simulink model "Buck_DCM_Model_eZdsp"  (R2020a)
settings: Solver=FixedStepAuto  StartTime=0.0  StopTime=inf  FixedStep=T  RelTol=1e-3
undefined symbols (not defined in the file): C, ILmax, Iumax, J, Kphi, L, Lu, rL, Ru, T, Ubat, Ucmax, wmax
libraries: c280xlib x16, simulink x4, c2833xlib x1
settings Model: SILPILModeSetting=veronly  ExtModeTrigDuration=8  Creator=Nguyen Tung  LastModifiedBy=Nguyen Tung
settings OptimizationCC: DefaultUnderspecifiedDataType=single  StrengthReduction=on  PassReuseOutputArgsAs=Individual arguments  MaxStackSize=1024  OptimizeBlockOrder=speed  OptimizationPriority=Speed  OptimizationCustomize=off  MultiThreadedLoops=on  DenormalBehavior=FlushToZero  EfficientTunableParamExpr=on
settings DebuggingCC: ParameterTunabilityLossMsg=error
settings HardwareCC: ProdBitPerChar=16  ProdBitPerInt=16  ProdBitPerPointer=32  ProdBitPerSizeT=32  ProdBitPerPtrDiffT=32  ProdLargestAtomicInteger=Integer  ProdLargestAtomicFloat=None  ProdWordSize=16  ProdLongLongMode=on  ProdHWDeviceType=Texas Instruments->C2000
settings SFSimCC: MATLABDynamicMemAlloc=off
settings RTWCC: SystemTargetFile=ert.tlc  HardwareBoard=TI Delfino F2833x  TLCOptions=-aInlineSetEventsForThisBaseRateFcn=TLC_FALSE -aSuppressMultiTaskScheduler=TLC_FALSE -aRateBasedStepFcn=1  TemplateMakefile=ert_default_tmf  GenerateReport=on  Toolchain=Texas Instruments Code Composer Studio (C2000)  BuildConfiguration=Faster Runs
settings CodeAppCC: ForceParamTrailComments=on  IgnoreCustomStorageClasses=off  OperatorAnnotations=on  SimulinkDataObjDesc=on  SFDataObjDesc=on  InsertBlockDesc=on
settings ERTTargetCC: CodeReplacementLibrary=TI C28x  SupportContinuousTime=on  ExtModeStaticAllocSize=10000

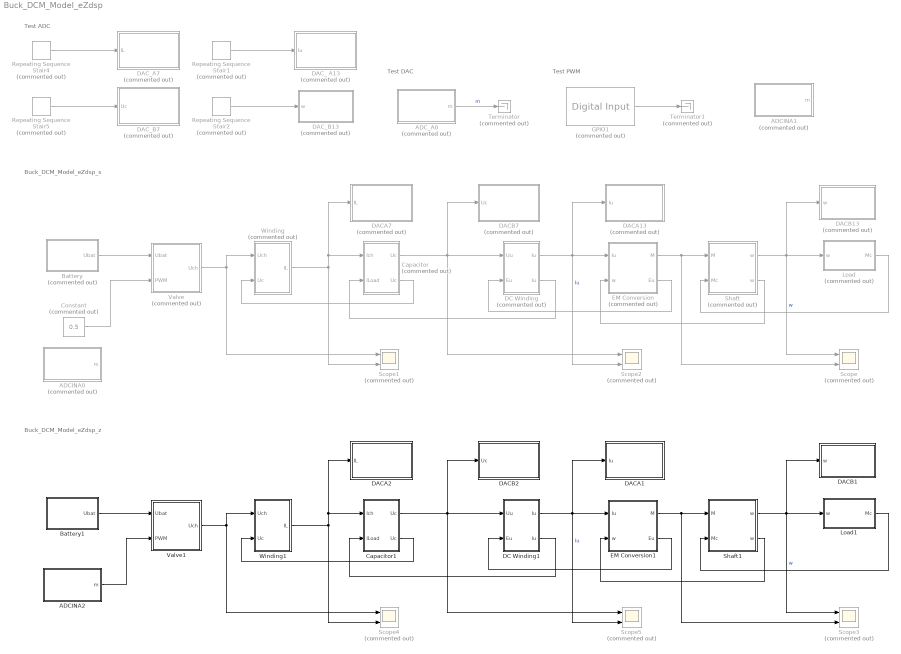
== system Buck_DCM_Model_eZdsp ==
  note: Buck_DCM_Model_eZdsp_s
  note: Test PWM
  note: Test DAC
  note: Test ADC
  note: Buck_DCM_Model_eZdsp_z
  ADCINA0 : Subsystem  Commented=on
  ADCINA1 : Subsystem  Commented=on
  ADCINA2 : Subsystem
  ADC_A0 : Subsystem  Commented=on
  Battery : Subsystem  Commented=on  AncestorBlock=simulink/REM/SE
      mask Display:
      | plot(0,0,100,100, 1.2*[50,57.68,60.77,63.08,64.97,66.58,68,69.26,70.4, 	71.42,72.36,78.28,80,78.28,72.36,71.42,70.4, 	69.26,68,66.58,64.97,63.08,60.77,57.68,50,42.32, 	39.23,36.92,35.03,33.42,32,30.74,29.6,28.58, 	27.64,21.72,20,21.72,27.64,28.58,29.6,30.74,32, 	33.42,35.03,36.92,39.23,42.32,50]-10, 1.2*[20,21,22,23,24,25,26,27,28,29,30,40,50,60,70,71,72, 	73,74,75,76,77,78,79,80,79,78,77,76,75,74,73,72, 	71,70,60,50,40,30,29,28,27,26,25,24,23,22,21,20]-10)
      | disp('ES')
  Battery1 : Subsystem  AncestorBlock=simulink/REM/SE
      mask Display:
      | plot(0,0,100,100, 1.2*[50,57.68,60.77,63.08,64.97,66.58,68,69.26,70.4, 	71.42,72.36,78.28,80,78.28,72.36,71.42,70.4, 	69.26,68,66.58,64.97,63.08,60.77,57.68,50,42.32, 	39.23,36.92,35.03,33.42,32,30.74,29.6,28.58, 	27.64,21.72,20,21.72,27.64,28.58,29.6,30.74,32, 	33.42,35.03,36.92,39.23,42.32,50]-10, 1.2*[20,21,22,23,24,25,26,27,28,29,30,40,50,60,70,71,72, 	73,74,75,76,77,78,79,80,79,78,77,76,75,74,73,72, 	71,70,60,50,40,30,29,28,27,26,25,24,23,22,21,20]-10)
      | disp('ES')
  Capacitor : Subsystem  Commented=on  AncestorBlock=simulink/REM/EA  mask(CM){}
      mask Display: plot(0,0,100,100,[10,10,90,90,10],[90,10,10,90,90], [10,90],[10,90])
  Capacitor1 : Subsystem  AncestorBlock=simulink/REM/EA  mask(CM){}
      mask Display: plot(0,0,100,100,[10,10,90,90,10],[90,10,10,90,90], [10,90],[10,90])
  Constant : Constant  Commented=on  Value=0.5
  DACA1 : Subsystem
  DACA13 : Subsystem  Commented=on
  DACA2 : Subsystem
  DACA7 : Subsystem  Commented=on
  DACB1 : Subsystem
  DACB13 : Subsystem  Commented=on
  DACB2 : Subsystem
  DACB7 : Subsystem  Commented=on
  DAC_ A13 : Subsystem  Commented=on
  DAC_A7 : Subsystem  Commented=on
  DAC_B13 : Subsystem  Commented=on
  DAC_B7 : Subsystem  Commented=on
  DC Winding : Subsystem  Commented=on  AncestorBlock=simulink/REM/EA  mask(CM){}
      mask Display: plot(0,0,100,100,[10,10,90,90,10],[90,10,10,90,90], [10,90],[10,90])
  DC Winding1 : Subsystem  AncestorBlock=simulink/REM/EA  mask(CM){}
      mask Display: plot(0,0,100,100,[10,10,90,90,10],[90,10,10,90,90], [10,90],[10,90])
  EM Conversion : Subsystem  Commented=on  AncestorBlock=simulink/REM/EC EM
      mask Display: plot(0,0,100,100, 1.4*[50,57.68,60.77,63.08,64.97,66.58,68,69.26,70.4, 	71.42,72.36,78.28,80,78.28,72.36,71.42,70.4, 	69.26,68,66.58,64.97,63.08,60.77,57.68,50,42.32, 	39.23,36.92,35.03,33.42,32,30.74,29.6,28.58, 	27.64,21.72,20,21.72,27.64,28.58,29.6,30.74,32, 	33.42,35.03,36.92,39.23,42.32,50]-20, 1.4*[20,21,22,23,24,25,26,27,28,29,30,40,50,60,70,71,72, 	73,74,75,76,77,78,79,80,79,78,77,76,75,74,73,72, 	71,70,60,50,40,30,29,28,27,26,25,24,23,22,21,20]-20)
  EM Conversion1 : Subsystem  AncestorBlock=simulink/REM/EC EM
      mask Display: plot(0,0,100,100, 1.4*[50,57.68,60.77,63.08,64.97,66.58,68,69.26,70.4, 	71.42,72.36,78.28,80,78.28,72.36,71.42,70.4, 	69.26,68,66.58,64.97,63.08,60.77,57.68,50,42.32, 	39.23,36.92,35.03,33.42,32,30.74,29.6,28.58, 	27.64,21.72,20,21.72,27.64,28.58,29.6,30.74,32, 	33.42,35.03,36.92,39.23,42.32,50]-20, 1.4*[20,21,22,23,24,25,26,27,28,29,30,40,50,60,70,71,72, 	73,74,75,76,77,78,79,80,79,78,77,76,75,74,73,72, 	71,70,60,50,40,30,29,28,27,26,25,24,23,22,21,20]-20)
  GPIO1 : c2833xlib/Digital Input  Commented=on  GPIO_Number=GPIO24~GPIO31  GPIO_Bit0=off  GPIO_Bit1=off  GPIO_Bit2=off  GPIO_Bit3=on  GPIO_Bit4=off  GPIO_Bit5=off  GPIO_Bit6=off  GPIO_Bit7=off  sampleTime=0.1  dataType=auto  GPIO_Bit0_Qualification=Sync to SYSCLKOUT  GPIO_Bit1_Qualification=Sync to SYSCLKOUT  GPIO_Bit2_Qualification=Sync to SYSCLKOUT  GPIO_Bit3_Qualification=Sync to SYSCLKOUT  GPIO_Bit4_Qualification=Sync to SYSCLKOUT  GPIO_Bit5_Qualification=Sync to SYSCLKOUT  GPIO_Bit6_Qualification=Sync to SYSCLKOUT  GPIO_Bit7_Qualification=Sync to SYSCLKOUT  Qualification_Period=-1
      settings: SourceProductBaseCode=TIC2000
  Load : Subsystem  Commented=on  AncestorBlock=simulink/REM/SE
      mask Display:
      | plot(0,0,100,100, 1.2*[50,57.68,60.77,63.08,64.97,66.58,68,69.26,70.4, 	71.42,72.36,78.28,80,78.28,72.36,71.42,70.4, 	69.26,68,66.58,64.97,63.08,60.77,57.68,50,42.32, 	39.23,36.92,35.03,33.42,32,30.74,29.6,28.58, 	27.64,21.72,20,21.72,27.64,28.58,29.6,30.74,32, 	33.42,35.03,36.92,39.23,42.32,50]-10, 1.2*[20,21,22,23,24,25,26,27,28,29,30,40,50,60,70,71,72, 	73,74,75,76,77,78,79,80,79,78,77,76,75,74,73,72, 	71,70,60,50,40,30,29,28,27,26,25,24,23,22,21,20]-10)
      | disp('MS')
  Load1 : Subsystem  AncestorBlock=simulink/REM/SE
      mask Display:
      | plot(0,0,100,100, 1.2*[50,57.68,60.77,63.08,64.97,66.58,68,69.26,70.4, 	71.42,72.36,78.28,80,78.28,72.36,71.42,70.4, 	69.26,68,66.58,64.97,63.08,60.77,57.68,50,42.32, 	39.23,36.92,35.03,33.42,32,30.74,29.6,28.58, 	27.64,21.72,20,21.72,27.64,28.58,29.6,30.74,32, 	33.42,35.03,36.92,39.23,42.32,50]-10, 1.2*[20,21,22,23,24,25,26,27,28,29,30,40,50,60,70,71,72, 	73,74,75,76,77,78,79,80,79,78,77,76,75,74,73,72, 	71,70,60,50,40,30,29,28,27,26,25,24,23,22,21,20]-10)
      | disp('MS')
  Repeating Sequence Stair1 : simulink/Sources/Repeating Sequence Stair  Commented=on  OutValues=[0 10 20 30 40 50 60].'  tsamp=T  OutMin=[]  OutMax=[]  OutDataTypeStr=double  OutputDataTypeScalingMode=double  OutDataType=fixdt(0,8)  ConRadixGroup=Best Precision: Vector-wise  OutScaling=2^-12
  Repeating Sequence Stair2 : simulink/Sources/Repeating Sequence Stair  Commented=on  OutValues=[0 10 20 30 40 50 60 70 80 90 100].'  tsamp=T  OutMin=[]  OutMax=[]  OutDataTypeStr=double  OutputDataTypeScalingMode=double  OutDataType=fixdt(0,8)  ConRadixGroup=Best Precision: Vector-wise  OutScaling=2^-12
  Repeating Sequence Stair4 : simulink/Sources/Repeating Sequence Stair  Commented=on  OutValues=[0 10 20 30 40 50 60].'  tsamp=T  OutMin=[]  OutMax=[]  OutDataTypeStr=double  OutputDataTypeScalingMode=double  OutDataType=fixdt(0,8)  ConRadixGroup=Best Precision: Vector-wise  OutScaling=2^-12
  Repeating Sequence Stair5 : simulink/Sources/Repeating Sequence Stair  Commented=on  OutValues=[0 50 100 150 200 250 300 350 400].'  tsamp=T  OutMin=[]  OutMax=[]  OutDataTypeStr=double  OutputDataTypeScalingMode=double  OutDataType=fixdt(0,8)  ConRadixGroup=Best Precision: Vector-wise  OutScaling=2^-12
  Scope{,1..5} (6 alike) : Scope  Commented=on  NumInputPorts=2
  Shaft : Subsystem  Commented=on  AncestorBlock=simulink/REM/EA  mask(CM){}
      mask Display: plot(0,0,100,100,[10,10,90,90,10],[90,10,10,90,90], [10,90],[10,90])
  Shaft1 : Subsystem  AncestorBlock=simulink/REM/EA  mask(CM){}
      mask Display: plot(0,0,100,100,[10,10,90,90,10],[90,10,10,90,90], [10,90],[10,90])
  Terminator : Terminator  Commented=on
  Terminator1 : Terminator  Commented=on
  Valve : Subsystem  Commented=on  AncestorBlock=simulink/REM/EC Elec  mask(Hacheur){}
      mask Display: plot(0,0,100,100,[10,10,90,90,10],[90,10,10,90,90])
  Valve1 : Subsystem  AncestorBlock=simulink/REM/EC Elec  mask(Hacheur){}
      mask Display: plot(0,0,100,100,[10,10,90,90,10],[90,10,10,90,90])
  Winding : Subsystem  Commented=on  AncestorBlock=simulink/REM/EA  mask(CM){}
      mask Display: plot(0,0,100,100,[10,10,90,90,10],[90,10,10,90,90], [10,90],[10,90])
  Winding1 : Subsystem  AncestorBlock=simulink/REM/EA  mask(CM){}
      mask Display: plot(0,0,100,100,[10,10,90,90,10],[90,10,10,90,90], [10,90],[10,90])
  wires:
  EM Conversion/2(Eu) -> DC Winding/2(Eu)
  DC Winding/1(Iu) -> Scope2/2, DACA13/1(Iu), EM Conversion/1(Iu)  "Iu"
  Capacitor/1(Uc) -> Scope2/1, DACB7/1(Uc), DC Winding/1(Uu)
  DC Winding/2("Iu ") -> Capacitor/2(ILoad)
  EM Conversion/1(M) -> Scope/2, Shaft/1(M)
  Valve/1(Uch) -> Winding/1(Uch), Scope1/1
  Battery/1(Ubat) -> Valve/1(Ubat)
  Load/1(Mc) -> Shaft/2(Mc)
  Shaft/2("w ") -> EM Conversion/2(w)
  Shaft/1(w) -> Scope/1, DACB13/1(w), Load/1(w)  "w"
  GPIO1/1 -> Terminator1/1
  ADC_A0/1(m) -> Terminator/1  "m"
  Repeating Sequence Stair4/1 -> DAC_A7/1(IL)
  Repeating Sequence Stair5/1 -> DAC_B7/1(Uc)
  Repeating Sequence Stair1/1 -> DAC_ A13/1(Iu)
  Repeating Sequence Stair2/1 -> DAC_B13/1(w)
  Constant/1 -> Valve/2(PWM)
  Capacitor/2("Uc ") -> Winding/2(Uc)
  Winding/1(IL) -> Scope1/2, Capacitor/1(Ich), DACA7/1(IL)
  Winding1/1(IL) -> Scope4/2, Capacitor1/1(Ich), DACA2/1(IL)
  DC Winding1/1(Iu) -> Scope5/2, DACA1/1(Iu), EM Conversion1/1(Iu)  "Iu"
  Battery1/1(Ubat) -> Valve1/1(Ubat)
  Capacitor1/2("Uc ") -> Winding1/2(Uc)
  Valve1/1(Uch) -> Winding1/1(Uch), Scope4/1
  EM Conversion1/1(M) -> Scope3/2, Shaft1/1(M)
  Shaft1/1(w) -> Scope3/1, DACB1/1(w), Load1/1(w)  "w"
  Load1/1(Mc) -> Shaft1/2(Mc)
  EM Conversion1/2(Eu) -> DC Winding1/2(Eu)
  Shaft1/2("w ") -> EM Conversion1/2(w)
  DC Winding1/2("Iu ") -> Capacitor1/2(ILoad)
  Capacitor1/1(Uc) -> Scope5/1, DACB2/1(Uc), DC Winding1/1(Uu)
  ADCINA2/1(m) -> Valve1/2(PWM)

== system Buck_DCM_Model_eZdsp/ADCINA0 ==
  ADC : c280xlib/ADC  useModule=A  useMode=Sequential  sourceSOC=Software  sourceSOC1=Software  sourceSOC2=ePWMxB  xint2_ADCSOC=31  Ts=T  dType=uint16  postInterrupt=off  numConversionsSingle=1  numConversionsDouble=1  conv0=ADCINA0  conv1=ADCINA1  conv2=ADCINA2  conv3=ADCINA3  conv4=ADCINA4  conv5=ADCINA5  conv6=ADCINA6  conv7=ADCINA7  conv8=ADCINB0  conv9=ADCINB1  conv10=ADCINB2  conv11=ADCINB3  conv12=ADCINB4  conv13=ADCINB5  conv14=ADCINB6  conv15=ADCINB7  convAB0=ADCINA0 and ADCINB0  convAB1=ADCINA1 and ADCINB1  convAB2=ADCINA2 and ADCINB2  convAB3=ADCINA3 and ADCINB3  convAB4=ADCINA4 and ADCINB4  convAB5=ADCINA5 and ADCINB5  convAB6=ADCINA6 and ADCINB6  convAB7=ADCINA7 and ADCINB7  convA0=ADCINA0  convA1=ADCINA1  convA2=ADCINA2  convA3=ADCINA3  convA4=ADCINA4  convA5=ADCINA5  convA6=ADCINA6  convA7=ADCINA7  convB0=ADCINB0  convB1=ADCINB1  convB2=ADCINB2  convB3=ADCINB3  convB4=ADCINB4  convB5=ADCINB5  convB6=ADCINB6  convB7=ADCINB7  c28xmultiPort=off  endma=off  chdma=1
      settings: SourceProductBaseCode=TIC2000
  Constant9 : Constant  Value=760
  Data Type Conversion8 : DataTypeConversion  OutMin=[0]  OutMax=[1]  OutDataTypeStr=single  SaturateOnIntegerOverflow=on
  Gain4 : Gain  Gain=1/3005
  Sum8 : Sum  Inputs=|+-
  m : Outport
  wires:
  Sum8/1 -> Gain4/1
  Constant9/1 -> Sum8/2
  ADC/1 -> Sum8/1
  Gain4/1 -> Data Type Conversion8/1
  Data Type Conversion8/1 -> m/1

== system Buck_DCM_Model_eZdsp/ADCINA1 ==
  ADC : c280xlib/ADC  useModule=A  useMode=Sequential  sourceSOC=Software  sourceSOC1=Software  sourceSOC2=ePWMxB  xint2_ADCSOC=31  Ts=T  dType=uint16  postInterrupt=off  numConversionsSingle=1  numConversionsDouble=1  conv0=ADCINA0  conv1=ADCINA1  conv2=ADCINA2  conv3=ADCINA3  conv4=ADCINA4  conv5=ADCINA5  conv6=ADCINA6  conv7=ADCINA7  conv8=ADCINB0  conv9=ADCINB1  conv10=ADCINB2  conv11=ADCINB3  conv12=ADCINB4  conv13=ADCINB5  conv14=ADCINB6  conv15=ADCINB7  convAB0=ADCINA0 and ADCINB0  convAB1=ADCINA1 and ADCINB1  convAB2=ADCINA2 and ADCINB2  convAB3=ADCINA3 and ADCINB3  convAB4=ADCINA4 and ADCINB4  convAB5=ADCINA5 and ADCINB5  convAB6=ADCINA6 and ADCINB6  convAB7=ADCINA7 and ADCINB7  convA0=ADCINA0  convA1=ADCINA1  convA2=ADCINA2  convA3=ADCINA3  convA4=ADCINA4  convA5=ADCINA5  convA6=ADCINA6  convA7=ADCINA7  convB0=ADCINB0  convB1=ADCINB1  convB2=ADCINB2  convB3=ADCINB3  convB4=ADCINB4  convB5=ADCINB5  convB6=ADCINB6  convB7=ADCINB7  c28xmultiPort=off  endma=off  chdma=1
      settings: SourceProductBaseCode=TIC2000
  Constant9 : Constant  Value=760
  Data Type Conversion8 : DataTypeConversion  OutMin=[0]  OutMax=[1]  OutDataTypeStr=single  SaturateOnIntegerOverflow=on
  Gain4 : Gain  Gain=1/3005
  Sum8 : Sum  Inputs=|+-
  m : Outport
  wires:
  Sum8/1 -> Gain4/1
  Constant9/1 -> Sum8/2
  ADC/1 -> Sum8/1
  Gain4/1 -> Data Type Conversion8/1
  Data Type Conversion8/1 -> m/1

== system Buck_DCM_Model_eZdsp/ADCINA2 ==
  ADC : c280xlib/ADC  useModule=A  useMode=Sequential  sourceSOC=Software  sourceSOC1=Software  sourceSOC2=ePWMxB  xint2_ADCSOC=31  Ts=T  dType=uint16  postInterrupt=off  numConversionsSingle=1  numConversionsDouble=1  conv0=ADCINA0  conv1=ADCINA1  conv2=ADCINA2  conv3=ADCINA3  conv4=ADCINA4  conv5=ADCINA5  conv6=ADCINA6  conv7=ADCINA7  conv8=ADCINB0  conv9=ADCINB1  conv10=ADCINB2  conv11=ADCINB3  conv12=ADCINB4  conv13=ADCINB5  conv14=ADCINB6  conv15=ADCINB7  convAB0=ADCINA0 and ADCINB0  convAB1=ADCINA1 and ADCINB1  convAB2=ADCINA2 and ADCINB2  convAB3=ADCINA3 and ADCINB3  convAB4=ADCINA4 and ADCINB4  convAB5=ADCINA5 and ADCINB5  convAB6=ADCINA6 and ADCINB6  convAB7=ADCINA7 and ADCINB7  convA0=ADCINA0  convA1=ADCINA1  convA2=ADCINA2  convA3=ADCINA3  convA4=ADCINA4  convA5=ADCINA5  convA6=ADCINA6  convA7=ADCINA7  convB0=ADCINB0  convB1=ADCINB1  convB2=ADCINB2  convB3=ADCINB3  convB4=ADCINB4  convB5=ADCINB5  convB6=ADCINB6  convB7=ADCINB7  c28xmultiPort=off  endma=off  chdma=1
      settings: SourceProductBaseCode=TIC2000
  Constant9 : Constant  Value=760
  Data Type Conversion8 : DataTypeConversion  OutMin=[0]  OutMax=[1]  OutDataTypeStr=single  SaturateOnIntegerOverflow=on
  Gain4 : Gain  Gain=1/3005
  Sum8 : Sum  Inputs=|+-
  m : Outport
  wires:
  Sum8/1 -> Gain4/1
  Constant9/1 -> Sum8/2
  ADC/1 -> Sum8/1
  Gain4/1 -> Data Type Conversion8/1
  Data Type Conversion8/1 -> m/1

== system Buck_DCM_Model_eZdsp/ADC_A0 ==
  ADC : c280xlib/ADC  useModule=A  useMode=Sequential  sourceSOC=Software  sourceSOC1=Software  sourceSOC2=ePWMxB  xint2_ADCSOC=31  Ts=T  dType=uint16  postInterrupt=off  numConversionsSingle=1  numConversionsDouble=1  conv0=ADCINA0  conv1=ADCINA1  conv2=ADCINA2  conv3=ADCINA3  conv4=ADCINA4  conv5=ADCINA5  conv6=ADCINA6  conv7=ADCINA7  conv8=ADCINB0  conv9=ADCINB1  conv10=ADCINB2  conv11=ADCINB3  conv12=ADCINB4  conv13=ADCINB5  conv14=ADCINB6  conv15=ADCINB7  convAB0=ADCINA0 and ADCINB0  convAB1=ADCINA1 and ADCINB1  convAB2=ADCINA2 and ADCINB2  convAB3=ADCINA3 and ADCINB3  convAB4=ADCINA4 and ADCINB4  convAB5=ADCINA5 and ADCINB5  convAB6=ADCINA6 and ADCINB6  convAB7=ADCINA7 and ADCINB7  convA0=ADCINA0  convA1=ADCINA1  convA2=ADCINA2  convA3=ADCINA3  convA4=ADCINA4  convA5=ADCINA5  convA6=ADCINA6  convA7=ADCINA7  convB0=ADCINB0  convB1=ADCINB1  convB2=ADCINB2  convB3=ADCINB3  convB4=ADCINB4  convB5=ADCINB5  convB6=ADCINB6  convB7=ADCINB7  c28xmultiPort=off  endma=off  chdma=1
      settings: SourceProductBaseCode=TIC2000
  Constant9 : Constant  Value=760
  Data Type Conversion8 : DataTypeConversion  OutMin=[0]  OutMax=[1]  OutDataTypeStr=single  SaturateOnIntegerOverflow=on
  Gain4 : Gain  Gain=1/3005
  Sum8 : Sum  Inputs=|+-
  m : Outport
  wires:
  Sum8/1 -> Gain4/1
  Constant9/1 -> Sum8/2
  ADC/1 -> Sum8/1
  Gain4/1 -> Data Type Conversion8/1
  Data Type Conversion8/1 -> m/1

== system Buck_DCM_Model_eZdsp/Battery ==
  Constant : Constant  Value=Ubat
  Ubat : Outport  InitialOutput=0  VectorParamsAs1DForOutWhenUnconnected=off
  wires:
  Constant/1 -> Ubat/1

== system Buck_DCM_Model_eZdsp/Battery1 ==
  Constant : Constant  Value=Ubat
  Ubat : Outport  InitialOutput=0  VectorParamsAs1DForOutWhenUnconnected=off
  wires:
  Constant/1 -> Ubat/1

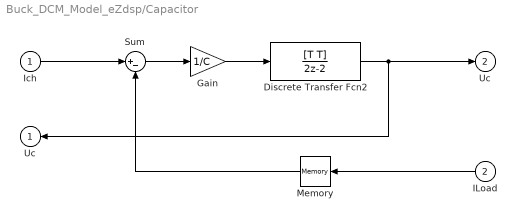
== system Buck_DCM_Model_eZdsp/Capacitor ==
  Ich : Inport
  ILoad : Inport  Port=2
  Discrete Transfer Fcn2 : DiscreteTransferFcn  Numerator=[T T]  Denominator=[2 -2]  SampleTime=T
  Gain : Gain  Gain=1/C
  Memory : Memory  LinearizeAsDelay=on
  Sum : Sum  Inputs=|+-
  Uc : Outport  InitialOutput=0  VectorParamsAs1DForOutWhenUnconnected=off
  "Uc " : Outport  Port=2  InitialOutput=0  VectorParamsAs1DForOutWhenUnconnected=off
  wires:
  Ich/1 -> Sum/1
  Sum/1 -> Gain/1
  Gain/1 -> Discrete Transfer Fcn2/1
  Discrete Transfer Fcn2/1 -> Uc/1, "Uc "/1
  ILoad/1 -> Memory/1
  Memory/1 -> Sum/2

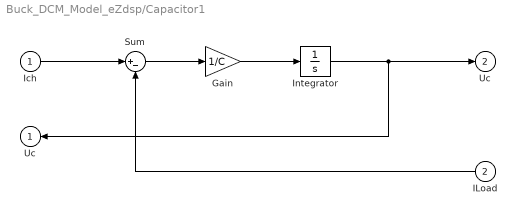
== system Buck_DCM_Model_eZdsp/Capacitor1 ==
  Ich : Inport
  ILoad : Inport  Port=2
  Gain : Gain  Gain=1/C
  Integrator : Integrator
  Sum : Sum  Inputs=|+-
  Uc : Outport  InitialOutput=0  VectorParamsAs1DForOutWhenUnconnected=off
  "Uc " : Outport  Port=2  InitialOutput=0  VectorParamsAs1DForOutWhenUnconnected=off
  wires:
  Ich/1 -> Sum/1
  Sum/1 -> Gain/1
  Gain/1 -> Integrator/1
  Integrator/1 -> Uc/1, "Uc "/1
  ILoad/1 -> Sum/2

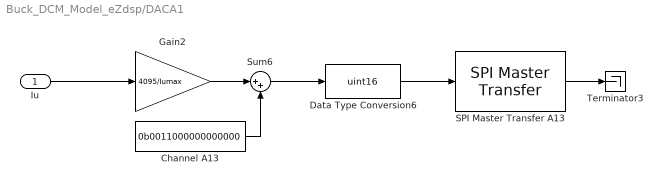
== system Buck_DCM_Model_eZdsp/DACA1 ==
  Iu : Inport
  Channel A13 : Constant  Value=0b0011000000000000
  Data Type Conversion6 : DataTypeConversion  OutDataTypeStr=uint16
  Gain2 : Gain  Gain=4095/Iumax
  SPI Master Transfer A13 : c280xlib/SPI Master Transfer  SPISelect=SPI_A  ClockPolarity=Falling_edge  ClockPhase=No_delay  SPIModule=uint32(0)  Mode=Master  BusSpeed=uint32(1000000)  FirstBitToTransfer=Most significant bit (MSB)  ClockMode=0  BlockFunction=Transfer  EnableRegisterAddress=off  RegisterAddress=0  OutputDataType=int8  OutputDataLength=1  DataBits=16  UseCustomSSPin=Explicit GPIO calls  ActiveLowSSPin=Active low  Pin=13
      settings: SourceProductBaseCode=TIC2000
  Sum6 : Sum  Inputs=|++
  Terminator3 : Terminator
  wires:
  Iu/1 -> Gain2/1
  Channel A13/1 -> Sum6/2
  Sum6/1 -> Data Type Conversion6/1
  SPI Master Transfer A13/1 -> Terminator3/1
  Gain2/1 -> Sum6/1
  Data Type Conversion6/1 -> SPI Master Transfer A13/1

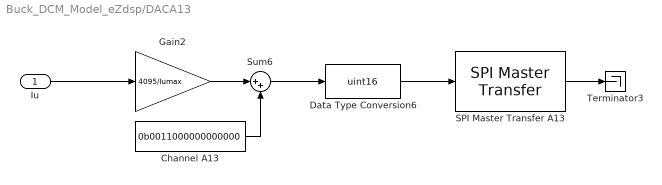
== system Buck_DCM_Model_eZdsp/DACA13 ==
  Iu : Inport
  Channel A13 : Constant  Value=0b0011000000000000
  Data Type Conversion6 : DataTypeConversion  OutDataTypeStr=uint16
  Gain2 : Gain  Gain=4095/Iumax
  SPI Master Transfer A13 : c280xlib/SPI Master Transfer  SPISelect=SPI_A  ClockPolarity=Falling_edge  ClockPhase=No_delay  SPIModule=uint32(0)  Mode=Master  BusSpeed=uint32(1000000)  FirstBitToTransfer=Most significant bit (MSB)  ClockMode=0  BlockFunction=Transfer  EnableRegisterAddress=off  RegisterAddress=0  OutputDataType=int8  OutputDataLength=1  DataBits=16  UseCustomSSPin=Explicit GPIO calls  ActiveLowSSPin=Active low  Pin=13
      settings: SourceProductBaseCode=TIC2000
  Sum6 : Sum  Inputs=|++
  Terminator3 : Terminator
  wires:
  Iu/1 -> Gain2/1
  Channel A13/1 -> Sum6/2
  Sum6/1 -> Data Type Conversion6/1
  SPI Master Transfer A13/1 -> Terminator3/1
  Gain2/1 -> Sum6/1
  Data Type Conversion6/1 -> SPI Master Transfer A13/1

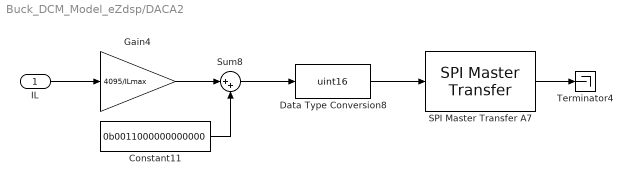
== system Buck_DCM_Model_eZdsp/DACA2 ==
  IL : Inport
  Constant11 : Constant  Value=0b0011000000000000
  Data Type Conversion8 : DataTypeConversion  OutDataTypeStr=uint16
  Gain4 : Gain  Gain=4095/ILmax
  SPI Master Transfer A7 : c280xlib/SPI Master Transfer  SPISelect=SPI_A  ClockPolarity=Falling_edge  ClockPhase=No_delay  SPIModule=uint32(0)  Mode=Master  BusSpeed=uint32(1000000)  FirstBitToTransfer=Most significant bit (MSB)  ClockMode=0  BlockFunction=Transfer  EnableRegisterAddress=off  RegisterAddress=0  OutputDataType=int8  OutputDataLength=1  DataBits=16  UseCustomSSPin=Explicit GPIO calls  ActiveLowSSPin=Active low  Pin=7
      settings: SourceProductBaseCode=TIC2000
  Sum8 : Sum  Inputs=|++
  Terminator4 : Terminator
  wires:
  Gain4/1 -> Sum8/1
  Constant11/1 -> Sum8/2
  Data Type Conversion8/1 -> SPI Master Transfer A7/1
  Sum8/1 -> Data Type Conversion8/1
  SPI Master Transfer A7/1 -> Terminator4/1
  IL/1 -> Gain4/1

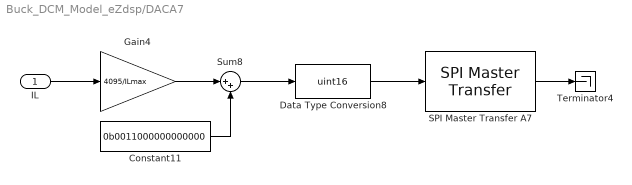
== system Buck_DCM_Model_eZdsp/DACA7 ==
  IL : Inport
  Constant11 : Constant  Value=0b0011000000000000
  Data Type Conversion8 : DataTypeConversion  OutDataTypeStr=uint16
  Gain4 : Gain  Gain=4095/ILmax
  SPI Master Transfer A7 : c280xlib/SPI Master Transfer  SPISelect=SPI_A  ClockPolarity=Falling_edge  ClockPhase=No_delay  SPIModule=uint32(0)  Mode=Master  BusSpeed=uint32(1000000)  FirstBitToTransfer=Most significant bit (MSB)  ClockMode=0  BlockFunction=Transfer  EnableRegisterAddress=off  RegisterAddress=0  OutputDataType=int8  OutputDataLength=1  DataBits=16  UseCustomSSPin=Explicit GPIO calls  ActiveLowSSPin=Active low  Pin=7
      settings: SourceProductBaseCode=TIC2000
  Sum8 : Sum  Inputs=|++
  Terminator4 : Terminator
  wires:
  Gain4/1 -> Sum8/1
  Constant11/1 -> Sum8/2
  Data Type Conversion8/1 -> SPI Master Transfer A7/1
  Sum8/1 -> Data Type Conversion8/1
  SPI Master Transfer A7/1 -> Terminator4/1
  IL/1 -> Gain4/1

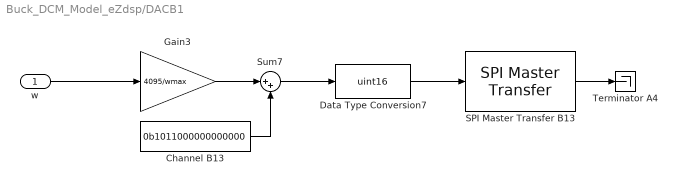
== system Buck_DCM_Model_eZdsp/DACB1 ==
  w : Inport
  Channel B13 : Constant  Value=0b1011000000000000
  Data Type Conversion7 : DataTypeConversion  OutDataTypeStr=uint16
  Gain3 : Gain  Gain=4095/wmax
  SPI Master Transfer B13 : c280xlib/SPI Master Transfer  SPISelect=SPI_A  ClockPolarity=Falling_edge  ClockPhase=No_delay  SPIModule=uint32(0)  Mode=Master  BusSpeed=uint32(1000000)  FirstBitToTransfer=Most significant bit (MSB)  ClockMode=0  BlockFunction=Transfer  EnableRegisterAddress=off  RegisterAddress=0  OutputDataType=int8  OutputDataLength=1  DataBits=16  UseCustomSSPin=Explicit GPIO calls  ActiveLowSSPin=Active low  Pin=13
      settings: SourceProductBaseCode=TIC2000
  Sum7 : Sum  Inputs=|++
  Terminator A4 : Terminator
  wires:
  Data Type Conversion7/1 -> SPI Master Transfer B13/1
  Gain3/1 -> Sum7/1
  w/1 -> Gain3/1
  Sum7/1 -> Data Type Conversion7/1
  SPI Master Transfer B13/1 -> Terminator A4/1
  Channel B13/1 -> Sum7/2

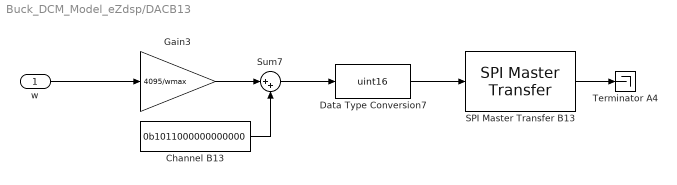
== system Buck_DCM_Model_eZdsp/DACB13 ==
  w : Inport
  Channel B13 : Constant  Value=0b1011000000000000
  Data Type Conversion7 : DataTypeConversion  OutDataTypeStr=uint16
  Gain3 : Gain  Gain=4095/wmax
  SPI Master Transfer B13 : c280xlib/SPI Master Transfer  SPISelect=SPI_A  ClockPolarity=Falling_edge  ClockPhase=No_delay  SPIModule=uint32(0)  Mode=Master  BusSpeed=uint32(1000000)  FirstBitToTransfer=Most significant bit (MSB)  ClockMode=0  BlockFunction=Transfer  EnableRegisterAddress=off  RegisterAddress=0  OutputDataType=int8  OutputDataLength=1  DataBits=16  UseCustomSSPin=Explicit GPIO calls  ActiveLowSSPin=Active low  Pin=13
      settings: SourceProductBaseCode=TIC2000
  Sum7 : Sum  Inputs=|++
  Terminator A4 : Terminator
  wires:
  Data Type Conversion7/1 -> SPI Master Transfer B13/1
  Gain3/1 -> Sum7/1
  w/1 -> Gain3/1
  Sum7/1 -> Data Type Conversion7/1
  SPI Master Transfer B13/1 -> Terminator A4/1
  Channel B13/1 -> Sum7/2

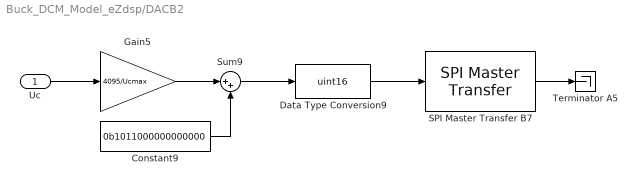
== system Buck_DCM_Model_eZdsp/DACB2 ==
  Uc : Inport
  Constant9 : Constant  Value=0b1011000000000000
  Data Type Conversion9 : DataTypeConversion  OutDataTypeStr=uint16
  Gain5 : Gain  Gain=4095/Ucmax
  SPI Master Transfer B7 : c280xlib/SPI Master Transfer  SPISelect=SPI_A  ClockPolarity=Falling_edge  ClockPhase=No_delay  SPIModule=uint32(0)  Mode=Master  BusSpeed=uint32(1000000)  FirstBitToTransfer=Most significant bit (MSB)  ClockMode=0  BlockFunction=Transfer  EnableRegisterAddress=off  RegisterAddress=0  OutputDataType=int8  OutputDataLength=1  DataBits=16  UseCustomSSPin=Explicit GPIO calls  ActiveLowSSPin=Active low  Pin=7
      settings: SourceProductBaseCode=TIC2000
  Sum9 : Sum  Inputs=|++
  Terminator A5 : Terminator
  wires:
  Constant9/1 -> Sum9/2
  Gain5/1 -> Sum9/1
  SPI Master Transfer B7/1 -> Terminator A5/1
  Sum9/1 -> Data Type Conversion9/1
  Data Type Conversion9/1 -> SPI Master Transfer B7/1
  Uc/1 -> Gain5/1

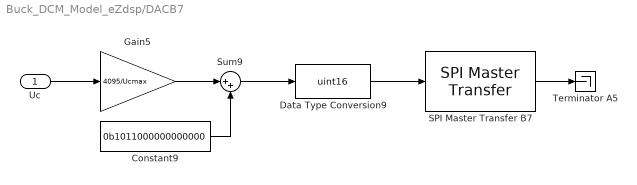
== system Buck_DCM_Model_eZdsp/DACB7 ==
  Uc : Inport
  Constant9 : Constant  Value=0b1011000000000000
  Data Type Conversion9 : DataTypeConversion  OutDataTypeStr=uint16
  Gain5 : Gain  Gain=4095/Ucmax
  SPI Master Transfer B7 : c280xlib/SPI Master Transfer  SPISelect=SPI_A  ClockPolarity=Falling_edge  ClockPhase=No_delay  SPIModule=uint32(0)  Mode=Master  BusSpeed=uint32(1000000)  FirstBitToTransfer=Most significant bit (MSB)  ClockMode=0  BlockFunction=Transfer  EnableRegisterAddress=off  RegisterAddress=0  OutputDataType=int8  OutputDataLength=1  DataBits=16  UseCustomSSPin=Explicit GPIO calls  ActiveLowSSPin=Active low  Pin=7
      settings: SourceProductBaseCode=TIC2000
  Sum9 : Sum  Inputs=|++
  Terminator A5 : Terminator
  wires:
  Constant9/1 -> Sum9/2
  Gain5/1 -> Sum9/1
  SPI Master Transfer B7/1 -> Terminator A5/1
  Sum9/1 -> Data Type Conversion9/1
  Data Type Conversion9/1 -> SPI Master Transfer B7/1
  Uc/1 -> Gain5/1

== system Buck_DCM_Model_eZdsp/DAC_ A13 ==
  Iu : Inport
  Channel A13 : Constant  Value=0b0011000000000000
  Data Type Conversion6 : DataTypeConversion  OutDataTypeStr=uint16
  Gain2 : Gain  Gain=4095/Iumax
  SPI Master Transfer A13 : c280xlib/SPI Master Transfer  SPISelect=SPI_A  ClockPolarity=Falling_edge  ClockPhase=No_delay  SPIModule=uint32(0)  Mode=Master  BusSpeed=uint32(1000000)  FirstBitToTransfer=Most significant bit (MSB)  ClockMode=0  BlockFunction=Transfer  EnableRegisterAddress=off  RegisterAddress=0  OutputDataType=int8  OutputDataLength=1  DataBits=16  UseCustomSSPin=Explicit GPIO calls  ActiveLowSSPin=Active low  Pin=13
      settings: SourceProductBaseCode=TIC2000
  Sum6 : Sum  Inputs=|++
  Terminator3 : Terminator
  wires:
  Iu/1 -> Gain2/1
  Channel A13/1 -> Sum6/2
  Sum6/1 -> Data Type Conversion6/1
  SPI Master Transfer A13/1 -> Terminator3/1
  Gain2/1 -> Sum6/1
  Data Type Conversion6/1 -> SPI Master Transfer A13/1

== system Buck_DCM_Model_eZdsp/DAC_A7 ==
  IL : Inport
  Constant11 : Constant  Value=0b0011000000000000
  Data Type Conversion8 : DataTypeConversion  OutDataTypeStr=uint16
  Gain4 : Gain  Gain=4095/ILmax
  SPI Master Transfer A7 : c280xlib/SPI Master Transfer  SPISelect=SPI_A  ClockPolarity=Falling_edge  ClockPhase=No_delay  SPIModule=uint32(0)  Mode=Master  BusSpeed=uint32(1000000)  FirstBitToTransfer=Most significant bit (MSB)  ClockMode=0  BlockFunction=Transfer  EnableRegisterAddress=off  RegisterAddress=0  OutputDataType=int8  OutputDataLength=1  DataBits=16  UseCustomSSPin=Explicit GPIO calls  ActiveLowSSPin=Active low  Pin=7
      settings: SourceProductBaseCode=TIC2000
  Sum8 : Sum  Inputs=|++
  Terminator4 : Terminator
  wires:
  Gain4/1 -> Sum8/1
  Constant11/1 -> Sum8/2
  Data Type Conversion8/1 -> SPI Master Transfer A7/1
  Sum8/1 -> Data Type Conversion8/1
  SPI Master Transfer A7/1 -> Terminator4/1
  IL/1 -> Gain4/1

== system Buck_DCM_Model_eZdsp/DAC_B13 ==
  w : Inport
  Channel B13 : Constant  Value=0b1011000000000000
  Data Type Conversion7 : DataTypeConversion  OutDataTypeStr=uint16
  Gain3 : Gain  Gain=4095/wmax
  SPI Master Transfer B13 : c280xlib/SPI Master Transfer  SPISelect=SPI_A  ClockPolarity=Falling_edge  ClockPhase=No_delay  SPIModule=uint32(0)  Mode=Master  BusSpeed=uint32(1000000)  FirstBitToTransfer=Most significant bit (MSB)  ClockMode=0  BlockFunction=Transfer  EnableRegisterAddress=off  RegisterAddress=0  OutputDataType=int8  OutputDataLength=1  DataBits=16  UseCustomSSPin=Explicit GPIO calls  ActiveLowSSPin=Active low  Pin=13
      settings: SourceProductBaseCode=TIC2000
  Sum7 : Sum  Inputs=|++
  Terminator A4 : Terminator
  wires:
  Data Type Conversion7/1 -> SPI Master Transfer B13/1
  Gain3/1 -> Sum7/1
  w/1 -> Gain3/1
  Sum7/1 -> Data Type Conversion7/1
  SPI Master Transfer B13/1 -> Terminator A4/1
  Channel B13/1 -> Sum7/2

== system Buck_DCM_Model_eZdsp/DAC_B7 ==
  Uc : Inport
  Constant9 : Constant  Value=0b1011000000000000
  Data Type Conversion9 : DataTypeConversion  OutDataTypeStr=uint16
  Gain5 : Gain  Gain=4095/Ucmax
  SPI Master Transfer B7 : c280xlib/SPI Master Transfer  SPISelect=SPI_A  ClockPolarity=Falling_edge  ClockPhase=No_delay  SPIModule=uint32(0)  Mode=Master  BusSpeed=uint32(1000000)  FirstBitToTransfer=Most significant bit (MSB)  ClockMode=0  BlockFunction=Transfer  EnableRegisterAddress=off  RegisterAddress=0  OutputDataType=int8  OutputDataLength=1  DataBits=16  UseCustomSSPin=Explicit GPIO calls  ActiveLowSSPin=Active low  Pin=7
      settings: SourceProductBaseCode=TIC2000
  Sum9 : Sum  Inputs=|++
  Terminator A5 : Terminator
  wires:
  Constant9/1 -> Sum9/2
  Gain5/1 -> Sum9/1
  SPI Master Transfer B7/1 -> Terminator A5/1
  Sum9/1 -> Data Type Conversion9/1
  Data Type Conversion9/1 -> SPI Master Transfer B7/1
  Uc/1 -> Gain5/1

== system Buck_DCM_Model_eZdsp/DC Winding ==
  Uu : Inport
  Eu : Inport  Port=2
  Discrete Transfer Fcn : DiscreteTransferFcn  Numerator=[T T]  Denominator=[(2*Lu+Ru*T) Ru*T-2*Lu]  SampleTime=T
  Memory : Memory
  Sum : Sum  Inputs=|+-
  Iu : Outport  InitialOutput=0  VectorParamsAs1DForOutWhenUnconnected=off
  "Iu " : Outport  Port=2  InitialOutput=0  VectorParamsAs1DForOutWhenUnconnected=off
  wires:
  Uu/1 -> Sum/1
  Sum/1 -> Discrete Transfer Fcn/1
  Discrete Transfer Fcn/1 -> "Iu "/1, Iu/1
  Eu/1 -> Memory/1
  Memory/1 -> Sum/2

== system Buck_DCM_Model_eZdsp/DC Winding1 ==
  Uu : Inport
  Eu : Inport  Port=2
  Sum : Sum  Inputs=|+-
  Transfer Fcn : TransferFcn  Denominator=[Lu Ru]
  Iu : Outport  InitialOutput=0  VectorParamsAs1DForOutWhenUnconnected=off
  "Iu " : Outport  Port=2  InitialOutput=0  VectorParamsAs1DForOutWhenUnconnected=off
  wires:
  Uu/1 -> Sum/1
  Sum/1 -> Transfer Fcn/1
  Transfer Fcn/1 -> "Iu "/1, Iu/1
  Eu/1 -> Sum/2

== system Buck_DCM_Model_eZdsp/EM Conversion ==
  Iu : Inport
  w : Inport  Port=2
  Gain : Gain  Gain=Kphi
  Gain1 : Gain  Gain=Kphi
  M : Outport  InitialOutput=0  VectorParamsAs1DForOutWhenUnconnected=off
  Eu : Outport  Port=2  InitialOutput=0  VectorParamsAs1DForOutWhenUnconnected=off
  wires:
  Iu/1 -> Gain/1
  Gain/1 -> M/1
  w/1 -> Gain1/1
  Gain1/1 -> Eu/1

== system Buck_DCM_Model_eZdsp/EM Conversion1 ==
  Iu : Inport
  w : Inport  Port=2
  Gain : Gain  Gain=Kphi
  Gain1 : Gain  Gain=Kphi
  M : Outport  InitialOutput=0  VectorParamsAs1DForOutWhenUnconnected=off
  Eu : Outport  Port=2  InitialOutput=0  VectorParamsAs1DForOutWhenUnconnected=off
  wires:
  Iu/1 -> Gain/1
  Gain/1 -> M/1
  w/1 -> Gain1/1
  Gain1/1 -> Eu/1

== system Buck_DCM_Model_eZdsp/Load ==
  w : Inport
  Load : Step  Time=5  After=0  SampleTime=T
  Terminator : Terminator
  Mc : Outport  InitialOutput=0  VectorParamsAs1DForOutWhenUnconnected=off
  wires:
  w/1 -> Terminator/1
  Load/1 -> Mc/1

== system Buck_DCM_Model_eZdsp/Load1 ==
  w : Inport
  Load : Step  Time=5  After=10  SampleTime=T
  Terminator : Terminator
  Mc : Outport  InitialOutput=0  VectorParamsAs1DForOutWhenUnconnected=off
  wires:
  w/1 -> Terminator/1
  Load/1 -> Mc/1

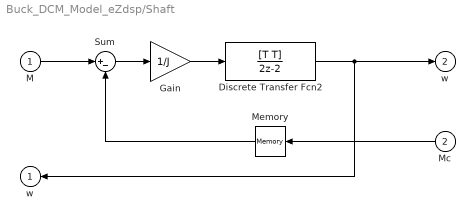
== system Buck_DCM_Model_eZdsp/Shaft ==
  M : Inport
  Mc : Inport  Port=2
  Discrete Transfer Fcn2 : DiscreteTransferFcn  Numerator=[T T]  Denominator=[2 -2]  SampleTime=T
  Gain : Gain  Gain=1/J
  Memory : Memory
  Sum : Sum  Inputs=|+-
  w : Outport  InitialOutput=0  VectorParamsAs1DForOutWhenUnconnected=off
  "w " : Outport  Port=2  InitialOutput=0  VectorParamsAs1DForOutWhenUnconnected=off
  wires:
  M/1 -> Sum/1
  Sum/1 -> Gain/1
  Gain/1 -> Discrete Transfer Fcn2/1
  Discrete Transfer Fcn2/1 -> "w "/1, w/1
  Mc/1 -> Memory/1
  Memory/1 -> Sum/2

== system Buck_DCM_Model_eZdsp/Shaft1 ==
  M : Inport
  Mc : Inport  Port=2
  Gain : Gain  Gain=1/J
  Integrator : Integrator
  Sum : Sum  Inputs=|+-
  w : Outport  InitialOutput=0  VectorParamsAs1DForOutWhenUnconnected=off
  "w " : Outport  Port=2  InitialOutput=0  VectorParamsAs1DForOutWhenUnconnected=off
  wires:
  M/1 -> Sum/1
  Sum/1 -> Gain/1
  Gain/1 -> Integrator/1
  Integrator/1 -> "w "/1, w/1
  Mc/1 -> Sum/2

== system Buck_DCM_Model_eZdsp/Valve ==
  Ubat : Inport
  PWM : Inport  Port=2
  Product : Product
  Uch : Outport  InitialOutput=0  VectorParamsAs1DForOutWhenUnconnected=off
  wires:
  Product/1 -> Uch/1
  Ubat/1 -> Product/1
  PWM/1 -> Product/2

== system Buck_DCM_Model_eZdsp/Valve1 ==
  Ubat : Inport
  PWM : Inport  Port=2
  Product : Product
  Uch : Outport  InitialOutput=0  VectorParamsAs1DForOutWhenUnconnected=off
  wires:
  Product/1 -> Uch/1
  Ubat/1 -> Product/1
  PWM/1 -> Product/2

== system Buck_DCM_Model_eZdsp/Winding ==
  Uch : Inport
  Uc : Inport  Port=2
  Discrete Transfer Fcn : DiscreteTransferFcn  Numerator=[T T]  Denominator=[(2*L+rL*T) rL*T-2*L]  SampleTime=T
  Memory : Memory
  Sum : Sum  Inputs=|+-
  IL : Outport  InitialOutput=0  VectorParamsAs1DForOutWhenUnconnected=off
  wires:
  Uch/1 -> Sum/1
  Sum/1 -> Discrete Transfer Fcn/1
  Discrete Transfer Fcn/1 -> IL/1
  Uc/1 -> Memory/1
  Memory/1 -> Sum/2

== system Buck_DCM_Model_eZdsp/Winding1 ==
  Uch : Inport
  Uc : Inport  Port=2
  Sum : Sum  Inputs=|+-
  Transfer Fcn : TransferFcn  Denominator=[L rL]
  IL : Outport  InitialOutput=0  VectorParamsAs1DForOutWhenUnconnected=off
  wires:
  Uch/1 -> Sum/1
  Sum/1 -> Transfer Fcn/1
  Transfer Fcn/1 -> IL/1
  Uc/1 -> Sum/2
